simulink model "UUV_simulink"  (R2021b)
settings: Solver=VariableStepAuto  StartTime=0.0  StopTime=10.0  RelTol=1e-3
values from neighbouring files (symbols this model uses):
  S0 = [0; 0; 0; 0; 0; 0]    [UUV_Simulink_Plots.m]    (also in UUV_simulink_Animation.m)
settings Model: Creator=Sushmanth Sai G  LastModifiedBy=Sushmanth Sai G

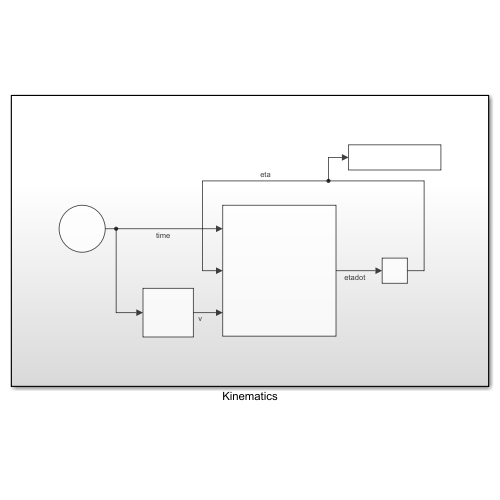
[thumbnail: Simulink's stored preview of the top-level diagram]
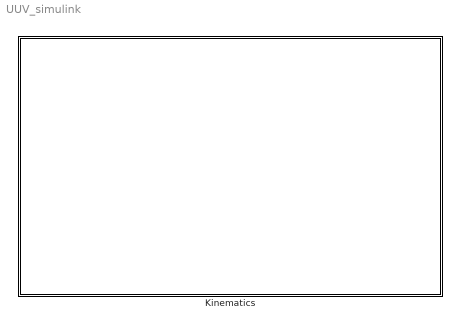
== system UUV_simulink ==
  Kinematics : Subsystem

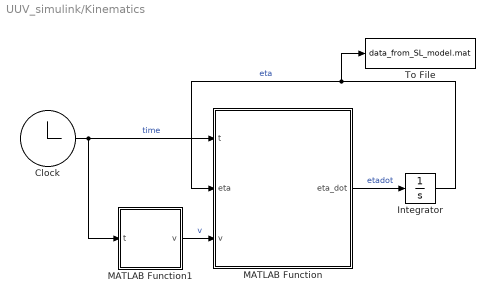
== system UUV_simulink/Kinematics ==
  Clock : Clock
  Integrator : Integrator  InitialCondition=S0
  MATLAB Function : MATLAB Function  TreatAsAtomicUnit=on
  MATLAB Function1 : MATLAB Function  TreatAsAtomicUnit=on
  To File : ToFile  Filename=data_from_SL_model.mat  MatrixName=eta
  wires:
  Clock/1 -> MATLAB Function/1(t), MATLAB Function1/1(t)  "time"
  Integrator/1 -> To File/1, MATLAB Function/2(eta)  "eta"
  MATLAB Function/1(eta_dot) -> Integrator/1  "etadot"
  MATLAB Function1/1(v) -> MATLAB Function/3(v)  "v"

== matlab function UUV_simulink/Kinematics/MATLAB Function ==
  data: t input; eta_dot output; eta input; v input
function eta_dot = V_P (t,eta,v)

phi = eta(4);
theta = eta(5);
psi = eta(6);

eta_dot = zeros(6,1);

Cpsi = [cos(psi) -sin(psi) 0
        sin(psi)  cos(psi) 0
        0          0       1];

Ctheta = [cos(theta)   0   sin(theta)
           0           1      0   
         -sin(theta)   0   cos(theta)];

Cphi = [1    0         0
        0 cos(phi) -sin(phi)
        0 sin(phi) cos(phi)];

J1 = Cpsi*Ctheta*Cphi;

J2= [1  sin(phi)*tan(theta)  cos(phi)*tan(theta)
     0      cos(phi)              -sin(phi)
     0 sin(phi)/cos(theta)   cos(phi)/cos(theta)]; 

J = [J1 zeros(3,3)
    zeros(3,3) J2];

eta_dot = J*v;

end

== matlab function UUV_simulink/Kinematics/MATLAB Function1 ==
  data: t input; v output
function v = f_v(t)
v = [0.5
     0
     0
     2*pi/10
     0
     0];
end
